simulink model "Traking_Control"  (R2018b)
settings: Solver=FixedStepDiscrete  StartTime=0.0  StopTime=Inf  FixedStep=0.005  RelTol=1e-3  EnableMultiTasking=on
undefined symbols (not defined in the file or in its folder): DiscIntNeverNeededParam, Send_GUIdata, Writer
libraries: simulink x4, c280xlib x4, c2833xlib x4, c2000lib x1, dspsrcs4 x1
settings Model: ExtModeTrigDuration=8  Creator=Administrator  LastModifiedBy=HP
settings OptimizationCC: DefaultUnderspecifiedDataType=single  EnhancedBackFolding=on  PassReuseOutputArgsAs=Individual arguments  MaxStackSize=512  OptimizeBlockOrder=speed  DifferentSizesBufferReuse=on  OptimizationCustomize=off
settings DebuggingCC: MultiTaskDSMMsg=none  ParameterTunabilityLossMsg=error
settings HardwareCC: ProdBitPerChar=16  ProdBitPerInt=16  ProdBitPerPointer=32  ProdBitPerSizeT=32  ProdBitPerPtrDiffT=32  ProdLargestAtomicInteger=Integer  ProdLargestAtomicFloat=None  ProdWordSize=16  ProdLongLongMode=on  ProdHWDeviceType=Texas Instruments->C2000
settings SFSimCC: MATLABDynamicMemAlloc=off
settings RTWCC: SystemTargetFile=ert.tlc  HardwareBoard=TI Delfino F2833x  TemplateMakefile=ert_default_tmf  GenerateReport=on  Toolchain=Texas Instruments Code Composer Studio (C2000)  IncludeHyperlinkInReport=on  LaunchReport=on  GenerateTraceInfo=on  GenerateTraceReport=on  GenerateTraceReportSl=on  GenerateTraceReportSf=on  GenerateTraceReportEml=on
settings CodeAppCC: ForceParamTrailComments=on  IgnoreCustomStorageClasses=off  OperatorAnnotations=on  SimulinkDataObjDesc=on  SFDataObjDesc=on  InsertBlockDesc=on
settings ERTTargetCC: CodeReplacementLibrary=TI C28x

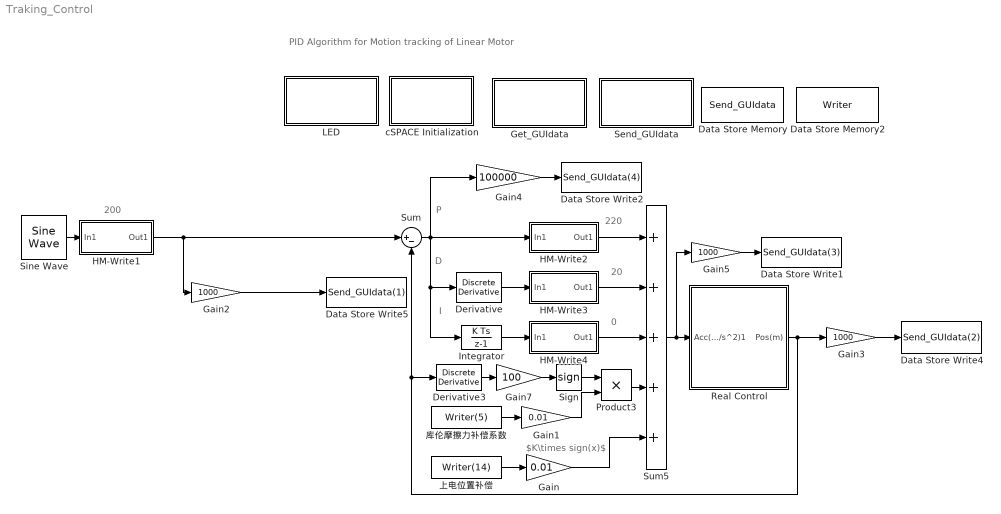
== system Traking_Control ==
  note: 20
  note: 220
  note: PID Algorithm for Motion tracking of Linear Motor
  note: D
  note: I
  note: 200
  note: P
  note: $K\times sign(x)$
  note: 0
  Data Store Memory : DataStoreMemory  DataStoreName=Send_GUIdata  ReadBeforeWriteMsg=warning  WriteAfterWriteMsg=warning  WriteAfterReadMsg=warning  InitialValue=zeros(1,10)  ShowAdditionalParam=off
  Data Store Memory2 : DataStoreMemory  DataStoreName=Writer  ReadBeforeWriteMsg=warning  WriteAfterWriteMsg=warning  WriteAfterReadMsg=warning  InitialValue=zeros(1,15)  ShowAdditionalParam=off  OutDataTypeStr=double
      settings: RTWStateStorageClass=ExportedGlobal
  Data Store Write1 : DataStoreWrite  DataStoreName=Send_GUIdata  DataStoreElements=Send_GUIdata(3)
  Data Store Write2 : DataStoreWrite  DataStoreName=Send_GUIdata  DataStoreElements=Send_GUIdata(4)
  Data Store Write4 : DataStoreWrite  DataStoreName=Send_GUIdata  DataStoreElements=Send_GUIdata(2)
  Data Store Write5 : DataStoreWrite  DataStoreName=Send_GUIdata  DataStoreElements=Send_GUIdata(1)
  Derivative : simulink/Discrete/Discrete Derivative  gainval=1.0  ICPrevScaledInput=0.0  OutMin=[]  OutMax=[]  OutDataType=sfix(16)  OutScaling=2^-10  DoSatur=off
  Derivative3 : simulink/Discrete/Discrete Derivative  gainval=1.0  ICPrevScaledInput=0.0  OutMin=[]  OutMax=[]  OutDataType=sfix(16)  OutScaling=2^-10  DoSatur=off
  Gain : Gain  Gain=0.01
  Gain1 : Gain  Gain=0.01
  Gain2 : Gain  Gain=1000
  Gain3 : Gain  Gain=1000
  Gain4 : Gain  Gain=100000
  Gain5 : Gain  Gain=1000
  Gain7 : Gain  Gain=100
  Get_GUIdata : Subsystem
      mask Display: disp('从上位机获取\n控制数据')
  HM-Write1 : Subsystem
  HM-Write2 : Subsystem
  HM-Write3 : Subsystem
  HM-Write4 : Subsystem
  Integrator : DiscreteIntegrator  SampleTime=-1  ICPrevOutput=DiscIntNeverNeededParam  ICPrevScaledInput=DiscIntNeverNeededParam
  LED : Subsystem  TreatAsAtomicUnit=on
      settings: RTWSystemCode=Nonreusable function
  Product3 : Product
  Real Control : Subsystem
      mask Display:
      | port_label('input',1,'Acc(m/s^2)','texmode','on');
      | port_label('output',1,'Pos(m)','texmode','on');
  Send_GUIdata : Subsystem  mask{VChoice=4}
      mask prompts: VChoice "Select a variant choice"
      mask help: 选择发送几路通道的数据，“4”：表示发送数据到上位机的通道1~4；“10”：表示发送数据到上位机的通道1~10
      mask init:
      | simulationStatus =  get_param(bdroot,'SimulationStatus');
      | 
      | % The active variant can only be modified at edit-time or very early during
      | % the simulink compile stage. 
      | 
      |     choice = get_param(gcb,'VChoice');
      |     vssBlk = [gcb, '/VariantSubsystem'];
      |     oldVariant = get_param(gcb,'OverrideUsingVariant');
      | 
      |     if strcmp(choice,'4')
      | 
      |         set_param(vssBlk, 'OverrideUsingVariant', 'Variant1');
      |     else
      | 
      |         set_param(vssBlk, 'OverrideUsingVariant', 'Variant2');
      |     end
      mask TypeOptions VChoice: 4 | 10
      mask Display: disp('发送数据\n到上位机显示')
  Sign : Signum
  Sine Wave : dspsrcs4/Sine Wave  Amplitude=1  Frequency=1/4  Phase=0  SampleMode=Discrete  OutComplex=Real  CompMethod=Trigonometric fcn  TableSize=Speed  SampleTime=5/1000  SamplesPerFrame=1  ResetState=Restart at time zero  OutputFrames=off  dataType=double  wordLen=16  udDataType=sfix(16)  fracBitsMode=Best precision  numFracBits=15  OutDataTypeStr=double  LastOutDataTypeStr=double
  Sum : Sum  Inputs=|+-
  Sum5 : Sum  Inputs=5
  cSPACE Initialization : Subsystem  Priority=0
      mask Display: disp('Initialize \ncSPACE');
  上电位置补偿 : DataStoreRead  DataStoreName=Writer  DataStoreElements=Writer(14)
  库伦摩擦力补偿系数 : DataStoreRead  DataStoreName=Writer  DataStoreElements=Writer(5)
  wires:
  Sum/1 -> HM-Write2/1(In1), Gain4/1, Integrator/1, Derivative/1
  Integrator/1 -> HM-Write4/1(In1)
  HM-Write2/1(Out1) -> Sum5/1
  HM-Write4/1(Out1) -> Sum5/3
  Sine Wave/1 -> HM-Write1/1(In1)
  Sum5/1 -> Gain5/1, Real Control/1(Acc(m/s^2)1)
  Derivative/1 -> HM-Write3/1(In1)
  HM-Write3/1(Out1) -> Sum5/2
  Gain7/1 -> Sign/1
  Real Control/1(Pos(m)) -> Gain3/1, Sum/2, Derivative3/1
  Gain1/1 -> Product3/2
  Sign/1 -> Product3/1
  库伦摩擦力补偿系数/1 -> Gain1/1
  Derivative3/1 -> Gain7/1
  Product3/1 -> Sum5/4
  上电位置补偿/1 -> Gain/1
  Gain/1 -> Sum5/5
  HM-Write1/1(Out1) -> Gain2/1, Sum/1
  Gain2/1 -> Data Store Write5/1
  Gain3/1 -> Data Store Write4/1
  Gain4/1 -> Data Store Write2/1
  Gain5/1 -> Data Store Write1/1

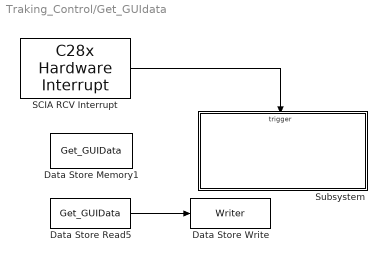
== system Traking_Control/Get_GUIdata ==
  Data Store Memory1 : DataStoreMemory  DataStoreName=Get_GUIData  ReadBeforeWriteMsg=warning  WriteAfterWriteMsg=warning  WriteAfterReadMsg=warning  InitialValue=zeros(1,15)  ShowAdditionalParam=off
      settings: RTWStateStorageClass=ExportedGlobal
  Data Store Read5 : DataStoreRead  DataStoreName=Get_GUIData
  Data Store Write : DataStoreWrite  DataStoreName=Writer
  SCIA RCV Interrupt : c2000lib/Scheduling/C28x Hardware Interrupt  irqnumbers=9  pienumbers=1  irqpriorities=1  irqpreempts=0  showinput=off  dspchiptype=C280X
      settings: SourceProductName=Embedded Coder Support Package for Texas Instruments C2000 Processors  SourceProductBaseCode=TIC2000
  Subsystem : Subsystem
      settings: PropExecContextOutsideSubsystem=on
  wires:
  SCIA RCV Interrupt/1 -> Subsystem/Trigger
  Data Store Read5/1 -> Data Store Write/1

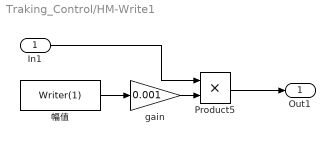
== system Traking_Control/HM-Write1 ==
  In1 : Inport
  Product5 : Product
  gain : Gain  Gain=0.001  OutDataTypeStr=double
  幅值 : DataStoreRead  DataStoreName=Writer  DataStoreElements=Writer(1)
  Out1 : Outport
  wires:
  In1/1 -> Product5/1
  Product5/1 -> Out1/1
  幅值/1 -> gain/1
  gain/1 -> Product5/2

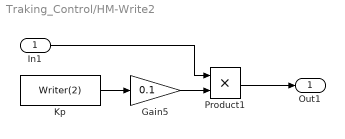
== system Traking_Control/HM-Write2 ==
  In1 : Inport
  Gain5 : Gain  Gain=0.1  OutDataTypeStr=double
  Kp : DataStoreRead  DataStoreName=Writer  DataStoreElements=Writer(2)
  Product1 : Product
  Out1 : Outport
  wires:
  In1/1 -> Product1/1
  Product1/1 -> Out1/1
  Gain5/1 -> Product1/2
  Kp/1 -> Gain5/1

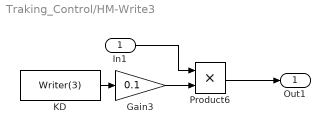
== system Traking_Control/HM-Write3 ==
  In1 : Inport
  Gain3 : Gain  Gain=0.1  OutDataTypeStr=double
  KD : DataStoreRead  DataStoreName=Writer  DataStoreElements=Writer(3)
  Product6 : Product
  Out1 : Outport
  wires:
  Gain3/1 -> Product6/2
  KD/1 -> Gain3/1
  Product6/1 -> Out1/1
  In1/1 -> Product6/1

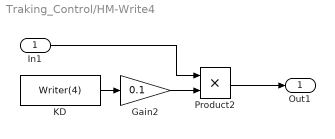
== system Traking_Control/HM-Write4 ==
  In1 : Inport
  Gain2 : Gain  Gain=0.1  OutDataTypeStr=double
  KD : DataStoreRead  DataStoreName=Writer  DataStoreElements=Writer(4)
  Product2 : Product
  Out1 : Outport
  wires:
  Product2/1 -> Out1/1
  KD/1 -> Gain2/1
  Gain2/1 -> Product2/2
  In1/1 -> Product2/1

== system Traking_Control/LED ==
  note: get
  CTC : simulink/Logic and Bit Operations/Compare To Constant  relop=<=  const=200  OutDataTypeStr=boolean
  Counter : simulink/Sources/Counter Limited  uplimit=400  tsamp=-1
  GPIO14 : c2833xlib/Digital Output  GPIO_Number=GPIO8~GPIO15  GPIO_Bit0=off  GPIO_BIT0_Toggle=off  GPIO_Bit1=off  GPIO_BIT1_Toggle=off  GPIO_Bit2=off  GPIO_BIT2_Toggle=off  GPIO_Bit3=off  GPIO_BIT3_Toggle=off  GPIO_Bit4=off  GPIO_BIT4_Toggle=off  GPIO_Bit5=off  GPIO_BIT5_Toggle=off  GPIO_Bit6=on  GPIO_BIT6_Toggle=off  GPIO_Bit7=off  GPIO_BIT7_Toggle=off
      settings: SourceProductName=Embedded Coder Support Package for Texas Instruments C2000 Processors  SourceProductBaseCode=TIC2000
  wires:
  Counter/1 -> CTC/1
  CTC/1 -> GPIO14/1

== system Traking_Control/Real Control ==
  Acc(m/s^2)1 : Inport
  Get Cart's Position : Subsystem  TreatAsAtomicUnit=on
      mask help:
      | 小车的位置分辨率:1um/脉冲
      | 位置单位：m
      settings: RTWSystemCode=Nonreusable function
      mask Display: disp('Get Position');
  "Set Cart's Acc " : Subsystem
      mask help: 将加速度通过数字电压转换成最终的模拟电压驱使小车移动
      mask Display:
      | disp('          SetAcc');
      | port_label('input', 1, 'Acc(m/s^2)');
  Pos(m) : Outport
  wires:
  Get Cart's Position/1(Pos(m)) -> Pos(m)/1
  Acc(m/s^2)1/1 -> "Set Cart's Acc "/1(In1)

== system Traking_Control/Send_GUIdata ==
  Data Store Read20 : DataStoreRead  DataStoreName=Send_GUIdata
  VariantSubsystem : Subsystem  VariantControlMode=Label  Variant=on  LabelModeActiveChoice=Variant1
  wires:
  Data Store Read20/1 -> VariantSubsystem/1(In1)

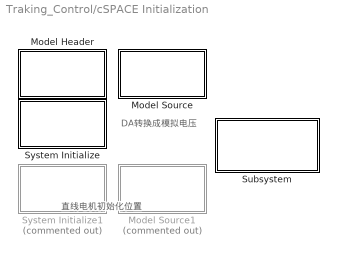
== system Traking_Control/cSPACE Initialization ==
  note: DA转换成模拟电压
  note: 直线电机初始化位置
  Model Header : Subsystem  mask(Model Header){ShowInLibBrowser=0}
      mask prompts: ShowInLibBrowser "Mask Parameter 1:"
      mask help: Add code to the model .h file
      settings: CopyFcn=cccopyfcn(gcb)  OpenFcn=ccopenfcn('Model Header')
      mask Help: eval('feval(''rtwprivate'',''rtwhelpview'',''rtw_model_header_block'')');
      mask Display: disp('Model\nHeader');
  Model Source : Subsystem  mask(Model Source){ShowInLibBrowser=0}
      mask prompts: ShowInLibBrowser "Mask Parameter 1:"
      mask help: Add code to the model .c file
      settings: CopyFcn=cccopyfcn(gcb)  OpenFcn=ccopenfcn('Model Source')
      mask Help: helpview([docroot '/toolbox/rtw/helptargets.map'], 'rtw_model_source_block');
      mask Display: disp('Model\nSource');
  Model Source1 : Subsystem  Commented=on  mask(Model Source){ShowInLibBrowser=0}
      mask prompts: ShowInLibBrowser "Mask Parameter 1:"
      mask help: Add code to the model .c file
      settings: CopyFcn=cccopyfcn(gcb)  OpenFcn=ccopenfcn('Model Source')
      mask Help: eval('feval(''rtwprivate'',''rtwhelpview'',''rtw_model_source_block'')');
      mask Display: disp('Model\nSource');
  Subsystem : Subsystem  TreatAsAtomicUnit=on
      settings: RTWSystemCode=Nonreusable function
      mask Display: disp('Elmo驱动器IO复位')
  System Initialize : Subsystem  mask(System Initialize){ShowInLibBrowser=0}
      mask prompts: ShowInLibBrowser "Mask Parameter 1:"
      mask help: Add code to a systems Initialize function
      settings: CopyFcn=cccopyfcn(gcb)  OpenFcn=ccopenfcn('System Initialize Function')
      mask Help: helpview([docroot '/toolbox/rtw/helptargets.map'], 'rtw_sys_initialize_block');
      mask Display: disp('System\nInitialize');
  System Initialize1 : Subsystem  Commented=on  mask(System Initialize){ShowInLibBrowser=0}
      mask prompts: ShowInLibBrowser "Mask Parameter 1:"
      mask help: Add code to a systems Initialize function
      settings: CopyFcn=cccopyfcn(gcb)  OpenFcn=ccopenfcn('System Initialize Function')
      mask Help: eval('feval(''rtwprivate'',''rtwhelpview'',''rtw_sys_initialize_block'')');
      mask Display: disp('System\nInitialize');

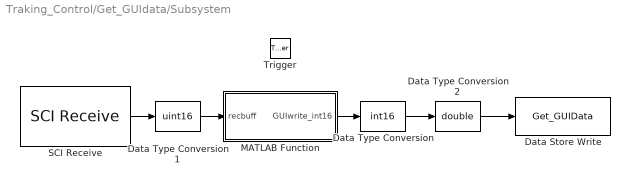
== system Traking_Control/Get_GUIdata/Subsystem ==
  Trigger : TriggerPort  TriggerType=function-call  VariantControl=Variant  PortDimensions=1
  Data Store Write : DataStoreWrite  DataStoreName=Get_GUIData
  Data Type Conversion : DataTypeConversion  OutDataTypeStr=int16
  Data Type Conversion1 : DataTypeConversion  OutDataTypeStr=uint16
  Data Type Conversion2 : DataTypeConversion  OutDataTypeStr=double
  MATLAB Function : MATLAB Function  TreatAsAtomicUnit=on
  SCI Receive : c280xlib/SCI Receive  sciModule=A  dataHead=''  dataTail=''  dataType=uint8  dataDim=32  initValue=0  errOption=Output the last received value  errValue=0  sampleTime=-1  outputStatus=off  postInterrupt=on  numFifo=16
      settings: SourceProductName=Embedded Coder Support Package for Texas Instruments C2000 Processors  SourceProductBaseCode=TIC2000
  wires:
  SCI Receive/1 -> Data Type Conversion1/1
  MATLAB Function/1(GUIwrite_int16) -> Data Type Conversion/1
  Data Type Conversion1/1 -> MATLAB Function/1(recbuff)
  Data Type Conversion/1 -> Data Type Conversion2/1
  Data Type Conversion2/1 -> Data Store Write/1

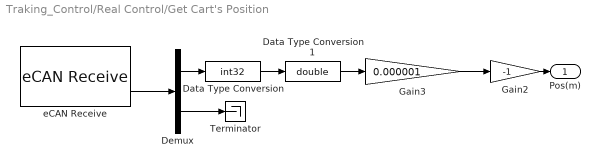
== system Traking_Control/Real Control/Get Cart's Position ==
  Data Type Conversion : DataTypeConversion  OutDataTypeStr=int32
  Data Type Conversion1 : DataTypeConversion  OutDataTypeStr=double
  Demux : Demux  Outputs=2
  Gain2 : Gain  Gain=-1
  Gain3 : Gain  Gain=0.000001
  Terminator : Terminator
  eCAN Receive : c280xlib/eCAN Receive  chipFamily=C280x  useModule=eCAN_A  mailboxNo=0  messageID=1  messageType=Standard (11-bit identifier)  sampleTime=-1  dataType=uint32  initValue=0  outputMessageLength=off  outputMessageTimeStamp=off  postInterrupt=off  interruptLine=0
      settings: SourceProductName=Embedded Coder Support Package for Texas Instruments C2000 Processors  SourceProductBaseCode=TIC2000
  Pos(m) : Outport
  wires:
  eCAN Receive/2 -> Demux/1
  Demux/1 -> Data Type Conversion/1
  Data Type Conversion/1 -> Data Type Conversion1/1
  Demux/2 -> Terminator/1
  Gain3/1 -> Gain2/1
  Gain2/1 -> Pos(m)/1
  Data Type Conversion1/1 -> Gain3/1

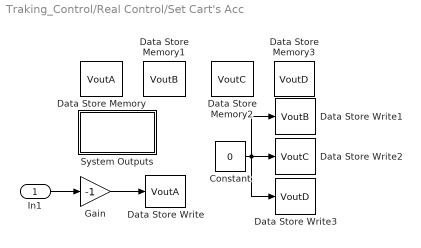
== system Traking_Control/Real Control/Set Cart's Acc  ==
  In1 : Inport
  Constant : Constant  Value=0
  Data Store Memory : DataStoreMemory  DataStoreName=VoutA  ReadBeforeWriteMsg=warning  WriteAfterWriteMsg=warning  WriteAfterReadMsg=warning  ShowAdditionalParam=off
      settings: RTWStateStorageClass=ExportedGlobal
  Data Store Memory1 : DataStoreMemory  DataStoreName=VoutB  ReadBeforeWriteMsg=warning  WriteAfterWriteMsg=warning  WriteAfterReadMsg=warning  ShowAdditionalParam=off
      settings: RTWStateStorageClass=ExportedGlobal
  Data Store Memory2 : DataStoreMemory  DataStoreName=VoutC  ReadBeforeWriteMsg=warning  WriteAfterWriteMsg=warning  WriteAfterReadMsg=warning  ShowAdditionalParam=off
      settings: RTWStateStorageClass=ExportedGlobal
  Data Store Memory3 : DataStoreMemory  DataStoreName=VoutD  ReadBeforeWriteMsg=warning  WriteAfterWriteMsg=warning  WriteAfterReadMsg=warning  ShowAdditionalParam=off
      settings: RTWStateStorageClass=ExportedGlobal
  Data Store Write : DataStoreWrite  DataStoreName=VoutA
  Data Store Write1 : DataStoreWrite  DataStoreName=VoutB
  Data Store Write2 : DataStoreWrite  DataStoreName=VoutC
  Data Store Write3 : DataStoreWrite  DataStoreName=VoutD
  Gain : Gain  Gain=-1
  System Outputs : Subsystem  mask(System Outputs){ShowInLibBrowser=0}
      mask prompts: ShowInLibBrowser "Mask Parameter 1:"
      mask help: Add code to a systems Outputs function
      settings: CopyFcn=cccopyfcn(gcb)  OpenFcn=ccopenfcn('System Outputs Function')
      mask Help: helpview([docroot '/toolbox/rtw/helptargets.map'], 'rtw_sys_outputs_block');
      mask Display: disp('System\nOutputs');
  wires:
  Constant/1 -> Data Store Write3/1, Data Store Write2/1, Data Store Write1/1
  In1/1 -> Gain/1
  Gain/1 -> Data Store Write/1

== system Traking_Control/Send_GUIdata/VariantSubsystem ==
  note: 1) Add Subsystem or Model blocks as valid variant choices.
      | 2) You cannot connect blocks at this level. At simulation, connectivity is automatically
      | determined, based on the active variant and port name matching.
  In1 : Inport
  Send10 : Subsystem  TreatAsAtomicUnit=on  VariantControl=Variant2
      settings: RTWSystemCode=Nonreusable function
  Srnd4 : Subsystem  TreatAsAtomicUnit=on  VariantControl=Variant1
      settings: RTWSystemCode=Nonreusable function

== system Traking_Control/cSPACE Initialization/Model Header ==

== system Traking_Control/cSPACE Initialization/Model Source ==

== system Traking_Control/cSPACE Initialization/Model Source1 ==

== system Traking_Control/cSPACE Initialization/Subsystem ==
  note: Elmo IO复位
  note: 28035 复位
  Constant : Constant
  Digital Output34 : c2833xlib/Digital Output  GPIO_Number=GPIO32~GPIO39  GPIO_Bit0=off  GPIO_BIT0_Toggle=off  GPIO_Bit1=off  GPIO_BIT1_Toggle=off  GPIO_Bit2=on  GPIO_BIT2_Toggle=off  GPIO_Bit3=off  GPIO_BIT3_Toggle=off  GPIO_Bit4=off  GPIO_BIT4_Toggle=off  GPIO_Bit5=off  GPIO_BIT5_Toggle=off  GPIO_Bit6=off  GPIO_BIT6_Toggle=off  GPIO_Bit7=off  GPIO_BIT7_Toggle=off
      settings: SourceProductName=Embedded Coder Support Package for Texas Instruments C2000 Processors  SourceProductBaseCode=TIC2000
  Digital Output35 : c2833xlib/Digital Output  GPIO_Number=GPIO32~GPIO39  GPIO_Bit0=off  GPIO_BIT0_Toggle=off  GPIO_Bit1=off  GPIO_BIT1_Toggle=off  GPIO_Bit2=off  GPIO_BIT2_Toggle=off  GPIO_Bit3=on  GPIO_BIT3_Toggle=off  GPIO_Bit4=off  GPIO_BIT4_Toggle=off  GPIO_Bit5=off  GPIO_BIT5_Toggle=off  GPIO_Bit6=off  GPIO_BIT6_Toggle=off  GPIO_Bit7=off  GPIO_BIT7_Toggle=off
      settings: SourceProductName=Embedded Coder Support Package for Texas Instruments C2000 Processors  SourceProductBaseCode=TIC2000
  Digital Output36 : c2833xlib/Digital Output  GPIO_Number=GPIO32~GPIO39  GPIO_Bit0=off  GPIO_BIT0_Toggle=off  GPIO_Bit1=off  GPIO_BIT1_Toggle=off  GPIO_Bit2=off  GPIO_BIT2_Toggle=off  GPIO_Bit3=off  GPIO_BIT3_Toggle=off  GPIO_Bit4=on  GPIO_BIT4_Toggle=off  GPIO_Bit5=off  GPIO_BIT5_Toggle=off  GPIO_Bit6=off  GPIO_BIT6_Toggle=off  GPIO_Bit7=off  GPIO_BIT7_Toggle=off
      settings: SourceProductName=Embedded Coder Support Package for Texas Instruments C2000 Processors  SourceProductBaseCode=TIC2000
  Step : Step  Time=0.5  SampleTime=0.005
  wires:
  Constant/1 -> Digital Output35/1, Digital Output36/1
  Step/1 -> Digital Output34/1

== system Traking_Control/cSPACE Initialization/System Initialize ==

== system Traking_Control/cSPACE Initialization/System Initialize1 ==

== system Traking_Control/Real Control/Set Cart's Acc /System Outputs ==

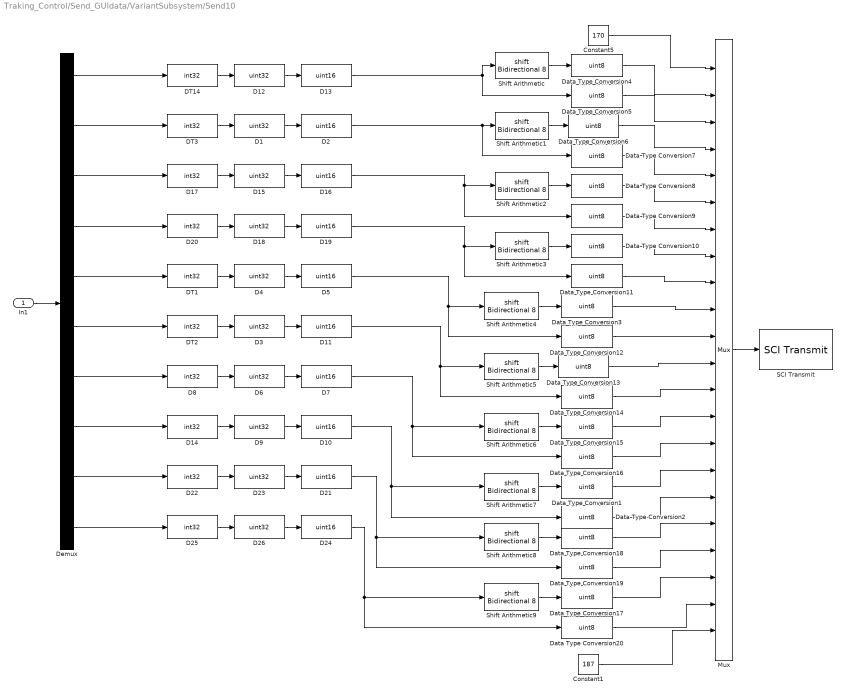
== system Traking_Control/Send_GUIdata/VariantSubsystem/Send10 ==
  In1 : Inport
  Constant1 : Constant  Value=187  OutDataTypeStr=uint8
  Constant5 : Constant  Value=170  OutDataTypeStr=uint8
  D{1,3..4,6,9,12,15,18,23,26} (10 alike) : DataTypeConversion  OutDataTypeStr=uint32
  D{2,5,7,10..11,13,16,19,21,24} (10 alike) : DataTypeConversion  OutDataTypeStr=uint16
  D{8,14,17,20,22,25} (6 alike) : DataTypeConversion  OutDataTypeStr=int32
  DT{1..3,14} (4 alike) : DataTypeConversion  OutDataTypeStr=int32
  Data Type Conversion{1..20} (20 alike) : DataTypeConversion  OutDataTypeStr=uint8
  Demux : Demux  Outputs=10
  Mux : Mux  Inputs=22
  SCI Transmit : c280xlib/SCI Transmit  sciModule=A  dataHead=''  dataTail=''  postInterrupt=on  numFifo=16
      settings: SourceProductName=Embedded Coder Support Package for Texas Instruments C2000 Processors
  Shift Arithmetic{,1..9} (10 alike) : ArithShift  BitShiftNumber=8
  wires:
  Demux/10 -> D25/1
  Demux/9 -> D22/1
  In1/1 -> Demux/1
  Demux/1 -> DT14/1
  Data Type Conversion11/1 -> Mux/9
  D12/1 -> D13/1
  Data Type Conversion9/1 -> Mux/7
  DT3/1 -> D1/1
  DT14/1 -> D12/1
  Shift Arithmetic2/1 -> Data Type Conversion8/1
  Data Type Conversion7/1 -> Mux/5
  Shift Arithmetic/1 -> Data Type Conversion4/1
  D15/1 -> D16/1
  D20/1 -> D18/1
  Data Type Conversion8/1 -> Mux/6
  D17/1 -> D15/1
  D18/1 -> D19/1
  D2/1 -> Shift Arithmetic1/1, Data Type Conversion7/1
  Data Type Conversion4/1 -> Mux/2
  Shift Arithmetic3/1 -> Data Type Conversion10/1
  Constant5/1 -> Mux/1
  Data Type Conversion6/1 -> Mux/4
  D19/1 -> Data Type Conversion11/1, Shift Arithmetic3/1
  Shift Arithmetic1/1 -> Data Type Conversion6/1
  Data Type Conversion5/1 -> Mux/3
  Mux/1 -> SCI Transmit/1
  Demux/4 -> D20/1
  D1/1 -> D2/1
  Demux/2 -> DT3/1
  Data Type Conversion10/1 -> Mux/8
  D16/1 -> Data Type Conversion9/1, Shift Arithmetic2/1
  Demux/3 -> D17/1
  D13/1 -> Data Type Conversion5/1, Shift Arithmetic/1
  D5/1 -> Data Type Conversion12/1, Shift Arithmetic4/1
  Data Type Conversion1/1 -> Mux/16
  Data Type Conversion12/1 -> Mux/11
  Shift Arithmetic5/1 -> Data Type Conversion13/1
  D10/1 -> Shift Arithmetic7/1, Data Type Conversion2/1
  Data Type Conversion13/1 -> Mux/12
  Shift Arithmetic7/1 -> Data Type Conversion1/1
  Data Type Conversion3/1 -> Mux/10
  D11/1 -> Data Type Conversion14/1, Shift Arithmetic5/1
  Data Type Conversion15/1 -> Mux/14
  Shift Arithmetic4/1 -> Data Type Conversion3/1
  Data Type Conversion14/1 -> Mux/13
  Shift Arithmetic6/1 -> Data Type Conversion15/1
  Data Type Conversion16/1 -> Mux/15
  Data Type Conversion2/1 -> Mux/17
  Demux/6 -> DT2/1
  D3/1 -> D11/1
  Demux/8 -> D14/1
  D9/1 -> D10/1
  D8/1 -> D6/1
  D14/1 -> D9/1
  D6/1 -> D7/1
  DT1/1 -> D4/1
  DT2/1 -> D3/1
  D4/1 -> D5/1
  Demux/7 -> D8/1
  D7/1 -> Shift Arithmetic6/1, Data Type Conversion16/1
  D22/1 -> D23/1
  D23/1 -> D21/1
  D26/1 -> D24/1
  D25/1 -> D26/1
  Demux/5 -> DT1/1
  Data Type Conversion20/1 -> Mux/21
  Data Type Conversion19/1 -> Mux/19
  Shift Arithmetic8/1 -> Data Type Conversion18/1
  Data Type Conversion18/1 -> Mux/18
  Shift Arithmetic9/1 -> Data Type Conversion17/1
  D24/1 -> Shift Arithmetic9/1, Data Type Conversion20/1
  Data Type Conversion17/1 -> Mux/20
  D21/1 -> Shift Arithmetic8/1, Data Type Conversion19/1
  Constant1/1 -> Mux/22

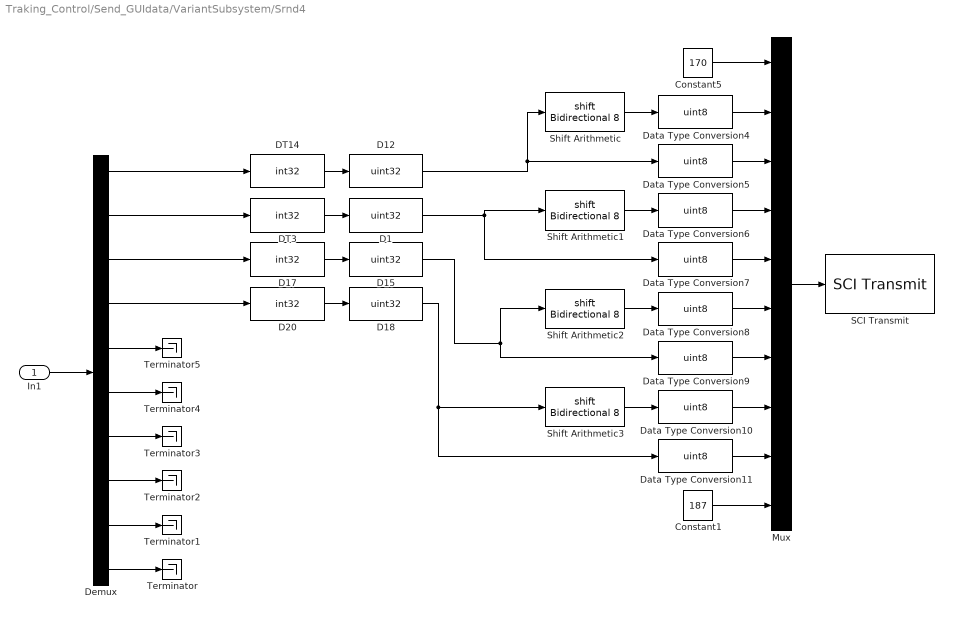
== system Traking_Control/Send_GUIdata/VariantSubsystem/Srnd4 ==
  In1 : Inport
  Constant1 : Constant  Value=187  OutDataTypeStr=uint8
  Constant5 : Constant  Value=170  OutDataTypeStr=uint8
  D{1,12,15,18} (4 alike) : DataTypeConversion  OutDataTypeStr=uint32
  D17 : DataTypeConversion  OutDataTypeStr=int32
  D20 : DataTypeConversion  OutDataTypeStr=int32
  DT14 : DataTypeConversion  OutDataTypeStr=int32
  DT3 : DataTypeConversion  OutDataTypeStr=int32
  Data Type Conversion{4..11} (8 alike) : DataTypeConversion  OutDataTypeStr=uint8
  Demux : Demux  Outputs=10
  Mux : Mux  Inputs=10
  SCI Transmit : c280xlib/SCI Transmit  sciModule=A  dataHead=''  dataTail=''  postInterrupt=on  numFifo=16
      settings: SourceProductName=Embedded Coder Support Package for Texas Instruments C2000 Processors
  Shift Arithmetic{,1..3} (4 alike) : ArithShift  BitShiftNumber=8
  Terminator{,1..5} (6 alike) : Terminator
  wires:
  In1/1 -> Demux/1
  Demux/3 -> D17/1
  Demux/1 -> DT14/1
  Demux/2 -> DT3/1
  Demux/4 -> D20/1
  Demux/10 -> Terminator/1
  Demux/9 -> Terminator1/1
  Demux/8 -> Terminator2/1
  Demux/7 -> Terminator3/1
  Demux/6 -> Terminator4/1
  Demux/5 -> Terminator5/1
  DT14/1 -> D12/1
  DT3/1 -> D1/1
  D17/1 -> D15/1
  D20/1 -> D18/1
  Data Type Conversion11/1 -> Mux/9
  Data Type Conversion9/1 -> Mux/7
  Shift Arithmetic2/1 -> Data Type Conversion8/1
  Data Type Conversion7/1 -> Mux/5
  D18/1 -> Data Type Conversion11/1, Shift Arithmetic3/1
  D1/1 -> Data Type Conversion7/1, Shift Arithmetic1/1
  Shift Arithmetic/1 -> Data Type Conversion4/1
  Data Type Conversion8/1 -> Mux/6
  Constant1/1 -> Mux/10
  Data Type Conversion4/1 -> Mux/2
  Shift Arithmetic3/1 -> Data Type Conversion10/1
  Data Type Conversion6/1 -> Mux/4
  Constant5/1 -> Mux/1
  Mux/1 -> SCI Transmit/1
  D15/1 -> Data Type Conversion9/1, Shift Arithmetic2/1
  D12/1 -> Shift Arithmetic/1, Data Type Conversion5/1
  Data Type Conversion5/1 -> Mux/3
  Data Type Conversion10/1 -> Mux/8
  Shift Arithmetic1/1 -> Data Type Conversion6/1

== matlab function Traking_Control/Get_GUIdata/Subsystem/MATLAB Function ==
  data: recbuff input; GUIwrite_int16 output
function GUIwrite_int16 = fcn(recbuff)
    GUIwrite_int16=[0 0 0 0 0 0 0 0 0 0 0 0 0 0 0];
    GUIwrite_int16(1)= recbuff(2)*256+recbuff(3);
    GUIwrite_int16(2)= recbuff(4)*256+recbuff(5);
    GUIwrite_int16(3)= recbuff(6)*256+recbuff(7);
    GUIwrite_int16(4)= recbuff(8)*256+recbuff(9);
    GUIwrite_int16(5)= recbuff(10)*256+recbuff(11);
    GUIwrite_int16(6)= recbuff(12)*256+recbuff(13);
    GUIwrite_int16(7)= recbuff(14)*256+recbuff(15);
    GUIwrite_int16(8)= recbuff(16)*256+recbuff(17);
    GUIwrite_int16(9)= recbuff(18)*256+recbuff(19);
    GUIwrite_int16(10)= recbuff(20)*256+recbuff(21);
    GUIwrite_int16(11)= recbuff(22)*256+recbuff(23);
    GUIwrite_int16(12)= recbuff(24)*256+recbuff(25);
    GUIwrite_int16(13)= recbuff(26)*256+recbuff(27);
    GUIwrite_int16(14)= recbuff(28)*256+recbuff(29);
    GUIwrite_int16(15)= recbuff(30)*256+recbuff(31);
end
